simulink model "EngineDynamometer"  (R2025a)
settings: configuration reference "EngDynoVariable" (kept outside this file)
model workspace (MAT data in the model file):
  DynOperatingPts : timeseries (value not decoded)
undefined symbols (not defined in the file): CiDynoMaxTurboSpd, CiDynoSSSpdCmd, CiDynoSSTrqCmd, DynoResultsBlock, EnvAbsPrs, EnvAirTemp, EnvRair, ExhCamPhaseCmd, InjPw, IntkCamPhaseCmd, Line, PlntEngAfrStoich, PlntEngCps, PlntEngNCyl, PlntEngSinj, PlntEngVd, si, si0, SiDynoMaxTurboSpd, SiDynoOpenLoopEngSpdCmdPts, SiDynoOpenLoopExhCamPhsCmdPts, SiDynoOpenLoopIntCamPhsCmdPts, SiDynoOpenLoopLambdaCmdPts, SiDynoOpenLoopMaxMAP, SiDynoOpenLoopSpkDeltaCmdPts, SiDynoOpenLoopSteadyStateWaitLimit, SiDynoOpenLoopTpCmdPts, SiDynoOpenLoopWAPCmdPts, SiDynoSSSpdCmd, SiDynoSSTrqCmd, SiDynoSSWaitLim, SpkAdv, ThrPosPctCmd, WgAreaPctCmd
libraries: autolibutils x4, autolibpowerinfoutils x1, simulink x1
(part 3 of 3)

== matlab function EngineDynamometer/Performance Monitor/Waitbar/Function-Call Subsystem/Waitbar ==
  data: FracComplete input
function ShowWaitBar(FracComplete)
coder.extrinsic('waitbar', 'figure', 'findall'); 
h = findall(0, 'Type', 'figure', 'Tag', 'DynamometerWaitbarFig');
if ~isempty(h)
    waitbar(FracComplete, h(1));
end

== stateflow chart EngineDynamometer/Performance Monitor/CheckToStop/Chart ==
  state Run
    during:
    doStop=false;
    state TrqCommand [parallel]
      settings: executionOrder=1
      state TrqCmd
        exit: time0 = time;
      state TrqCmdConst
        during:
        dTimeA = time-time0;
      (default) -> TrqCmd
      TrqCmd -> TrqCmdConst : [abs(trqCmd-trqCmd_1) <= 1]
      TrqCmdConst -> TrqCmd : [abs(trqCmd-trqCmd_1) > 1]
    state TrqDifference [parallel]
      settings: executionOrder=2
      state TrqDif
        exit: time00 = time;
      state TrqDifConst
        during:
        dTimeB = time-time00;
      (default) -> TrqDif
      TrqDif -> TrqDifConst : [abs(trqCmd-trq) >= 2]
      TrqDifConst -> TrqDif : [abs(trqCmd-trq) < 2]
    state TrqActual [parallel]
      settings: executionOrder=3
      state TrqDifChange
        exit: time000 = time;
      state TrqDifChConst
        during:
        dTimeC = time-time000;
      (default) -> TrqDifChange
      TrqDifChange -> TrqDifChConst : [abs(trq-trq_1) <= 1]
      TrqDifChConst -> TrqDifChange : [abs(trq-trq_1) > 1]
  state Stop
    entry:
    coder.extrinsic('message','RecalibrateSIController')
    RecalibrateSIController('', 'StopMsg')
    during:
    doStop=true;
  (default) -> Run
  Run -> Stop : [dTimeA>300&&dTimeB>300&&dTimeC>300]
  data: time input; trq input; trqCmd input; trqCmd_1 input; trq_1 input; dTimeA local =0; dTimeB local =0; dTimeC local =0; time0 local; time00 local; time000 local; doStop output

== stateflow chart EngineDynamometer/Dynamometer Control/Calibrate Throttle and Wastegate/TPP and WAP Calibration Controller ==
  state CalibrationLoop [parallel]
    settings: executionOrder=2
    state TorqueControl [group]
      state WaitForSteadyState
        en:
        LogDataTrigger = false;
        during:
        TrqCmd = max(EngTrq, MinTrqCmd);
      state GotoMaxTrq
        en:
        LoadLoggedCtrlValues(2)
        during:
        TrqCmd = max(EngTrq, MinTrqCmd);
      state LogData
        en:
        LogDataTrigger = true;
      state CompleteTorquePoint
        en:
        EngTrq0 = EngTrq;
        FracComplete = min(max((EngSpdIndex - 1 + (TrqCmd - MinTrqCmd)/(MaxTrqCmd - MinTrqCmd))/numel(EngSpdBpts), FracComplete), 1);
        EngTrqOvershoot = false;
      state IncreaseTrqCmd
        en:
        LogDataTrigger = false;
        TrqCmd = TrqCmd + MinTrqStep;
      WaitForSteadyState -> (junction 1632) [order 2] : after(1, sec)
          | [(EngTrq - EngTrq0) > MaxTrqStep && SteadyStateFlag]
          | {DecreaseCtrlStep;
          | DecreaseCtrl;
          | EngTrqOvershoot = true;
          | MaxTrqReached = false;}
      (junction 1632) -> (junction 1639)
      WaitForSteadyState -> GotoMaxTrq [order 1] : [MaxTrqReached && ...
          | (EngTrq - EngTrq0) < MaxTrqStep &&...
          |  SteadyStateFlag]
      GotoMaxTrq -> (junction 1622) : after(1, sec)[SteadyStateFlag]
      (junction 1639) -> WaitForSteadyState
      (junction 1638) -> (junction 1639) : {IncreaseCtrl;}
      (junction 1624) -> WaitForSteadyState [order 2] : {LogCtrlValues(2);
          | IncreaseCtrl;}
      WaitForSteadyState -> CompleteTorquePoint [order 3] : [MinCtrlStepSizeReached]
          | {IncreaseCtrlStep;}
      WaitForSteadyState -> (junction 1640) [order 4] : after(1, sec)[SteadyStateFlag]
      (junction 1624) -> (junction 1622) [order 1] : [MaxTrqReached]
      (junction 1622) -> IncreaseTrqCmd [order 2]
      LogData -> (junction 1624) : after(0.01, sec)
      (junction 1637) -> (junction 1638) : {IncreaseCtrlStep;}
      (junction 1630) -> (junction 1637) [order 2]
      (junction 1623) -> (junction 1638) : {DecreaseCtrlStep;}
      (junction 1640) -> (junction 1630) [order 1] : [(EngTrq - EngTrq0) < MinTrqStep]
      (junction 1630) -> (junction 1623) [order 1] : [EngTrqOvershoot]
      (junction 1640) -> CompleteTorquePoint [order 2]
      CompleteTorquePoint -> LogData
      IncreaseTrqCmd -> CompleteTorquePoint : after(0.01, sec)
    state NewEngSpd [group]
      state AboveMinTrq
        during:
        TrqCmd = max(EngTrq, MinTrqCmd);
        MaxTrqReached = false;
      state BelowMinTrq
        during:
        MaxTrqReached = false;
        TrqCmd = max(EngTrq, MinTrqCmd);
      AboveMinTrq -> BelowMinTrq [order 1] : [EngTrq < MinTrqCmd - MinTrqStep...
          |  && ~MinCtrlStepSizeReached]
          | {DecreaseCtrlStep;
          | IncreaseCtrl;}
      BelowMinTrq -> AboveMinTrq [order 1] : [EngTrq > MinTrqCmd]
          | {DecreaseCtrlStep;
          | DecreaseCtrl;}
      (junction 1645) -> AboveMinTrq : {IncreaseCtrlStep;
          | DecreaseCtrl;}
      AboveMinTrq -> (junction 1670) [order 2] : after(1, sec)[SteadyStateFlag]
      (junction 1658) -> BelowMinTrq : {IncreaseCtrl;}
      BelowMinTrq -> (junction 1655) [order 2] : after(1, sec)[SteadyStateFlag]
      (junction 1670) -> (junction 1645) [order 2]
      (junction 1655) -> (junction 1658) [order 2]
      (junction 1670) -> (junction 1668) [order 1] : [MinCtrlStepSizeReached]
      (junction 1655) -> (junction 1659) [order 1] : [abs(EngTrq - MinTrqCmd) < MinTrqStep...
          | || MaxTrqReached]
      (junction 1668) -> (junction 1659)
    state Stop
      en:
      StopCmd = true;
    state GetMotoringTorque [group]
      state SetMotoringTorque
        en:
        TrqCmd = 0;
        CutOffFuel = 1;
      state LogMotoringData
        en:
        LogDataTrigger = true;
      state SetMinTrq
        en:
        TrqCmd = MinTrqCmd;
        CutOffFuel = 0;
        LogDataTrigger = false;
      SetMotoringTorque -> LogMotoringData : after(1, sec)[SteadyStateFlag]
      LogMotoringData -> SetMinTrq : after(0.01, sec)
    (default) -> (junction 1672) : {
        | EngSpdIndex = 0;
        | LoggedTPP = [0;0];
        | LoggedWAP = [0;0];
        | FracComplete = 0;
        | StartCtrl;
        | }
    (junction 1622) -> (junction 1672) [order 1] : [FracComplete >= ...
        | EngSpdIndex/numel(EngSpdBpts)]
    (junction 1672) -> BelowMinTrq [order 2] : {EngSpdIndex = EngSpdIndex + 1;
        | EngSpd = EngSpdBpts(EngSpdIndex);
        | LogDataTrigger = false;
        | ResetCtrl;
        | LoadLoggedCtrlValues(1); }
    (junction 1672) -> Stop [order 1] : [EngSpdIndex >= numel(EngSpdBpts)]
    (junction 1659) -> SetMotoringTorque : {LogCtrlValues(1);}
    SetMinTrq -> CompleteTorquePoint : after(1, sec)[SteadyStateFlag]
  state StartCtrl [function]
    (default) -> (junction 1687) : {
        | TPP = 5;
        | WAP = 100;
        | MaxCtrlStepSize = 5;
        | CtrlStepSize = 0.1;
        | LogCtrlValues(1)
        | LogCtrlValues(2)
        | }
  state DecreaseCtrl [function]
    (default) -> (junction 1442)
    (junction 1442) -> (junction 1439) [order 1] : [WAP < 100]
    (junction 1442) -> (junction 1443) [order 2] : {TPP = max(TPP - CtrlStepSize, 0);
        | WAP = 100;}
    (junction 1439) -> (junction 1444) : {WAP = min(WAP + CtrlStepSize, 100);
        | TPP = 100;}
    (junction 1444) -> (junction 1443)
    (junction 1443) -> (junction 1445)
  state DecreaseCtrlStep [function]
    (default) -> (junction 1491) : {CtrlStepSize = CtrlStepSize/2;
        | MinCtrlStepSize = 0.01;}
    (junction 1491) -> (junction 1490) [order 1] : [MinCtrlStepSize > CtrlStepSize]
    (junction 1491) -> (junction 1487) [order 2]
    (junction 1490) -> (junction 1489) : {CtrlStepSize = MinCtrlStepSize;
        | MinCtrlStepSizeReached = true;}
    (junction 1489) -> (junction 1487)
    (junction 1487) -> (junction 1452)
  state LogCtrlValues(Idx) [function]
    (default) -> (junction 1526) : {LoggedTPP(Idx) = TPP; LoggedWAP(Idx) = WAP;}
  state ResetCtrl [function]
    (default) -> (junction 1437) : {
        | CtrlStepSize = 0.1;
        | MinCtrlStepSizeReached = false;
        | }
  state IncreaseCtrl [function]
    (default) -> (junction 1455)
    (junction 1455) -> (junction 1456) [order 1] : [TPP >= 100]
    (junction 1455) -> (junction 1457) [order 2] : {TPP = min(TPP + CtrlStepSize, 100);
        | WAP = 100;}
    (junction 1456) -> (junction 1458) : {WAP = max(WAP - CtrlStepSize, 0);
        | TPP = 100;}
    (junction 1458) -> (junction 1457)
    (junction 1457) -> (junction 1459)
  state IncreaseCtrlStep [function]
    (default) -> (junction 1466) : {CtrlStepSize = min(2*CtrlStepSize, MaxCtrlStepSize);
        | MinCtrlStepSizeReached = false;}
  state LoadLoggedCtrlValues(Idx) [function]
    (default) -> (junction 1511) : {TPP = LoggedTPP(Idx); WAP = LoggedWAP(Idx);}
  state CheckTrqLimit [parallel]
    settings: executionOrder=1
    state TrqBelowMax
      en:
      MaxTrqReached = false;
    state TrqAboveMax
      en:
      MaxTrqReached = true;
    (default) -> TrqBelowMax
    TrqBelowMax -> TrqAboveMax : [TurboSpd > MaxTurboSpd || EngTrq > MaxTrqCmd ...
        | || WAP <= 0]
    TrqAboveMax -> TrqBelowMax : [~MaxTrqReached]
  data: Idx function_input; Idx function_input; SteadyStateFlag input; EngSpd output; TrqCmd output; EngSpdBpts input; MinTrqStep input; MaxTrqStep input; MinTrqCmd input; EngSpdIndex local; LogDataTrigger output; StopCmd output; FracComplete output; TPP output size=[1,1]; EngTrq0 local; WAP output size=[1,1]; MaxTrqCmd input; MaxTurboSpd input; EngTrq input; TurboSpd input; MaxTrqReached local; CtrlStepSize local; MaxCtrlStepSize local; MinCtrlStepSizeReached local; EngTrqOvershoot local; LoggedTPP local size=[2,1]; LoggedWAP local size=[2,1]; CutOffFuel output

== stateflow chart EngineDynamometer/Dynamometer Control/Open Loop/Select Operating Point ==
  state Startup
    en:
    EngSpd = EngSpdCmdPts(Index);
    TpCmd = TpCmdPts(Index);
    WAPCmd =100.; %Start with WAP full open
    ICPCmd=ICPCmdPts(Index);
    ECPCmd=ECPCmdPts(Index);
    SPKCmd=SPKCmdPts(Index);
    LAMCmd=LAMCmdPts(Index);
    WAPLearn=true;
  state LimitMAP
    en:
    WAPLearn=true;
    du:
    WAPCmd = WAPCmd-0.025;
  state RevertOperatingPoint
    en:
    WAPLimit=WAPCmd;
    du:
    EngSpd = LastEngSpeed;
    TpCmd = LastTp;
    WAPCmd =LastWap;
  state WaitForSteadyState
    en:
    WAPLearn=false;
    EngSpd = EngSpdCmdPts(Index);
    TpCmd = TpCmdPts(Index);
    WAPCmd=WAPLimit;
    FracComplete = Index/TotNumPoints;
    LogDataTrigger = false;
  state LogData
    ex:
    LogDataTrigger = true;
  state SetNewValue
    en:
    Index = Index + 1;
    LastTp=TpCmd;
    LastEngSpeed=EngSpd;
    LastWap=WAPCmd;
  state Stop
    en:
    FracComplete = 1;
    StopCmd = true;
  (default) -> Startup : {
      | Index = 1;
      | StopCmd = false;
      | LogDataTrigger = false;
      | FracComplete = 0;
      | LastTp=mean(TpCmdPts);
      | LastEngSpeed=mean(EngSpdCmdPts);
      | LastWap=100.;
      | TotNumPoints = min([numel(EngSpdCmdPts) numel(TpCmdPts) numel(WAPCmdPts) numel(ICPCmdPts) numel(ECPCmdPts) numel(SPKCmdPts) numel(LAMCmdPts)]);
      | WAPLearn=false;
      | }
  (junction 124) -> Startup
  SetNewValue -> (junction 124) [order 1] : after(0.1,sec)[~SteadyStateFlag]
  (junction 126) -> Startup
  SetNewValue -> (junction 126) [order 2] : after(1.5,sec)
  Startup -> LimitMAP : after(5,sec)
  LimitMAP -> RevertOperatingPoint : [(WAPCmd<=WAPCmdPts(Index))||(MAP>=MaxMAP)||(WAPCmd<=0.05)]
  RevertOperatingPoint -> WaitForSteadyState : after(12, sec)
  WaitForSteadyState -> LogData [order 2] : after(SteadyStateWaitLimit, sec)
  (junction 73) -> SetNewValue [order 1] : [Index < numel(EngSpdCmdPts) || ...
      |  Index < numel(TpCmdPts) ||...
      |  Index < numel(WAPCmdPts)||...
      |  Index < numel(ICPCmdPts)||...
      |  Index < numel(ECPCmdPts)||...
      |  Index < numel(SPKCmdPts)||...
      |  Index < numel(LAMCmdPts)]
  LogData -> (junction 73) : after(0.01, sec)
  (junction 73) -> Stop [order 2]
  WaitForSteadyState -> LogData [order 1] : [SteadyStateFlag]
  data: SteadyStateFlag input; SteadyStateWaitLimit input; EngSpd output; EngSpdCmdPts input; TpCmdPts input; LogDataTrigger output; StopCmd output; FracComplete output; TotNumPoints local; TpCmd output; WAPCmd output; WAPCmdPts input; Index local; ICPCmdPts input; ECPCmdPts input; SPKCmdPts input; ICPCmd output; ECPCmd output; LAMCmd output; SPKCmd output; LAMCmdPts input; MAP input; WAPLimit local; LastTp local; LastEngSpeed local; LastWap local; WAPLearn output; MaxMAP input

== stateflow chart EngineDynamometer/Dynamometer Control/Calibration Controller/Fuel Calibration Controller ==
  state CalibrationLoop [parallel]
    settings: executionOrder=2
    state TorqueControl [group]
      state WaitForSteadyState
        en:
        LogDataTrigger = false;
        during:
        TrqCmd = max(EngTrq, MinTrqCmd);
      state GotoMaxTrq
        en:
        LoadLoggedCtrlValues(2)
        during:
        TrqCmd = max(EngTrq, MinTrqCmd);
      state LogData
        en:
        LogDataTrigger = true;
      state CompleteTorquePoint
        en:
        EngTrq0 = EngTrq;
        FracComplete = min(max((EngSpdIndex - 1 + (TrqCmd - MinTrqCmd)/(MaxTrqCmd - MinTrqCmd))/numel(EngSpdBpts), FracComplete), 1);
        EngTrqOvershoot = false;
      state IncreaseTrqCmd
        en:
        LogDataTrigger = false;
        TrqCmd = TrqCmd + MinTrqStep;
      WaitForSteadyState -> (junction 1701) [order 2] : after(1, sec)
          | [(EngTrq - EngTrq0) > MaxTrqStep && SteadyStateFlag]
          | {DecreaseCtrlStep;
          | DecreaseCtrl;
          | EngTrqOvershoot = true;
          | MaxTrqReached = false;}
      (junction 1701) -> (junction 1715)
      WaitForSteadyState -> GotoMaxTrq [order 1] : [MaxTrqReached && ...
          | (EngTrq - EngTrq0) < MaxTrqStep &&...
          |  SteadyStateFlag]
      GotoMaxTrq -> (junction 1733) : after(1, sec)[SteadyStateFlag]
      (junction 1715) -> WaitForSteadyState
      (junction 1760) -> (junction 1715) : {IncreaseCtrl;}
      (junction 1738) -> WaitForSteadyState [order 2] : {LogCtrlValues(2);
          | IncreaseCtrl;}
      WaitForSteadyState -> CompleteTorquePoint [order 3] : [MinCtrlStepSizeReached]
          | {IncreaseCtrlStep;}
      WaitForSteadyState -> (junction 1713) [order 4] : after(1, sec)[SteadyStateFlag]
      (junction 1738) -> (junction 1733) [order 1] : [MaxTrqReached]
      (junction 1733) -> IncreaseTrqCmd [order 2]
      LogData -> (junction 1738) : after(0.01, sec)
      (junction 1749) -> (junction 1760) : {IncreaseCtrlStep;}
      (junction 1744) -> (junction 1749) [order 2]
      (junction 1736) -> (junction 1760) : {DecreaseCtrlStep;}
      (junction 1713) -> (junction 1744) [order 1] : [(EngTrq - EngTrq0) < MinTrqStep]
      (junction 1744) -> (junction 1736) [order 1] : [EngTrqOvershoot]
      (junction 1713) -> CompleteTorquePoint [order 2]
      CompleteTorquePoint -> LogData
      IncreaseTrqCmd -> CompleteTorquePoint : after(0.01, sec)
    state NewEngSpd [group]
      state AboveMinTrq
        during:
        TrqCmd = max(EngTrq, MinTrqCmd);
        MaxTrqReached = false;
      state BelowMinTrq
        during:
        MaxTrqReached = false;
        TrqCmd = max(EngTrq, MinTrqCmd);
      AboveMinTrq -> BelowMinTrq [order 1] : [EngTrq < MinTrqCmd - MinTrqStep...
          |  && ~MinCtrlStepSizeReached]
          | {DecreaseCtrlStep;
          | IncreaseCtrl;}
      BelowMinTrq -> AboveMinTrq [order 1] : [EngTrq > MinTrqCmd]
          | {DecreaseCtrlStep;
          | DecreaseCtrl;}
      (junction 1734) -> AboveMinTrq : {IncreaseCtrlStep;
          | DecreaseCtrl;}
      AboveMinTrq -> (junction 1761) [order 2] : after(1, sec)[SteadyStateFlag]
      (junction 1714) -> BelowMinTrq : {IncreaseCtrl;}
      BelowMinTrq -> (junction 1740) [order 2] : after(1, sec)[SteadyStateFlag]
      (junction 1761) -> (junction 1734) [order 2]
      (junction 1740) -> (junction 1714) [order 2]
      (junction 1761) -> (junction 1762) [order 1] : [MinCtrlStepSizeReached]
      (junction 1740) -> (junction 1726) [order 1] : [abs(EngTrq - MinTrqCmd) < MinTrqStep...
          | || MaxTrqReached]
      (junction 1762) -> (junction 1726)
    state Stop
      en:
      StopCmd = true;
    state GetMotoringTorque [group]
      state SetMotoringTorque
        en:
        TrqCmd = 0;
        CutOffFuel = 1;
      state LogMotoringData
        en:
        LogDataTrigger = true;
      state SetMinTrq
        en:
        TrqCmd = MinTrqCmd;
        CutOffFuel = 0;
        LogDataTrigger = false;
      SetMotoringTorque -> LogMotoringData : after(1, sec)[SteadyStateFlag]
      LogMotoringData -> SetMinTrq : after(0.01, sec)
    (default) -> (junction 1706) : {
        | EngSpdIndex = 0;
        | LoggedFuelMass = [0;0];
        | FracComplete = 0;
        | StartCtrl;
        | }
    (junction 1733) -> (junction 1706) [order 1] : [FracComplete >= ...
        | EngSpdIndex/numel(EngSpdBpts)]
    (junction 1706) -> BelowMinTrq [order 2] : {EngSpdIndex = EngSpdIndex + 1;
        | EngSpd = EngSpdBpts(EngSpdIndex);
        | LogDataTrigger = false;
        | ResetCtrl;
        | LoadLoggedCtrlValues(1); }
    (junction 1706) -> Stop [order 1] : [EngSpdIndex >= numel(EngSpdBpts)]
    (junction 1726) -> SetMotoringTorque : {LogCtrlValues(1);}
    SetMinTrq -> CompleteTorquePoint : after(1, sec)[SteadyStateFlag]
  state StartCtrl [function]
    (default) -> (junction 1628) : {
        | MaxCtrlStepSize = 200*MinCtrlStepSize;
        | FuelMass = 500*MinCtrlStepSize;
        | CtrlStepSize = 10*MinCtrlStepSize;
        | LogCtrlValues(1)
        | LogCtrlValues(2)
        | }
  state DecreaseCtrl [function]
    (default) -> (junction 1445) : {FuelMass = FuelMass - CtrlStepSize;}
  state DecreaseCtrlStep [function]
    (default) -> (junction 1491) : {CtrlStepSize = CtrlStepSize/2;}
    (junction 1491) -> (junction 1490) [order 1] : [MinCtrlStepSize > CtrlStepSize]
    (junction 1491) -> (junction 1487) [order 2]
    (junction 1490) -> (junction 1489) : {CtrlStepSize = MinCtrlStepSize;
        | MinCtrlStepSizeReached = true;}
    (junction 1489) -> (junction 1487)
    (junction 1487) -> (junction 1452)
  state LogCtrlValues(Idx) [function]
    (default) -> (junction 1526) : {LoggedFuelMass(Idx) = FuelMass;}
  state ResetCtrl [function]
    (default) -> (junction 1437) : {
        | MinCtrlStepSizeReached = false;
        | CtrlStepSize = 10*MinCtrlStepSize;
        | }
  state IncreaseCtrl [function]
    (default) -> (junction 1554) : {FuelMass = FuelMass + CtrlStepSize;}
  state IncreaseCtrlStep [function]
    (default) -> (junction 1466) : {CtrlStepSize = min(2*CtrlStepSize, MaxCtrlStepSize);
        | MinCtrlStepSizeReached = false;}
  state LoadLoggedCtrlValues(Idx) [function]
    (default) -> (junction 1511) : {FuelMass = LoggedFuelMass(Idx);}
  state CheckTrqLimit [parallel]
    settings: executionOrder=1
    state TrqBelowMax
      en:
      MaxTrqReached = false;
    state TrqAboveMax
      en:
      MaxTrqReached = true;
    (default) -> TrqBelowMax : {MinAfr = 12;}
    TrqBelowMax -> TrqAboveMax : [TurboSpd > MaxTurboSpd || EngTrq > MaxTrqCmd ...
        | || Afr < MinAfr]
    TrqAboveMax -> TrqBelowMax : [~MaxTrqReached]
  data: Idx function_input; Idx function_input; SteadyStateFlag input; EngSpd output; TrqCmd output; EngSpdBpts input; MinTrqStep input; MaxTrqStep input; MinTrqCmd input; EngSpdIndex local; LogDataTrigger output; StopCmd output; FracComplete output; CutOffFuel output; FuelMass output; EngTrq0 local; MaxTrqCmd input; MaxTurboSpd input; MinCtrlStepSize input; EngTrq input; TurboSpd input; MaxTrqReached local; CtrlStepSize local; MaxCtrlStepSize local; MinCtrlStepSizeReached local; EngTrqOvershoot local; Afr input; MinAfr local; LoggedFuelMass local size=[2,1]
